simulink model "cyberAttack2"  (R2022b)
settings: Solver=VariableStepAuto  StartTime=0.0  StopTime=10  RelTol=1e-3
values from neighbouring files (symbols this model uses):
  attackTimeDelay = 0.1    [editor.m]
  attackTimeDelay1 = 0.1    [editor.m]
  CC_Kd = 0    [editor.m]
  CC_Ki = 150    [editor.m]
  CC_Kp = 0    [editor.m]
  enableObserver = 1    [editor.m]
  ICapacity_1 = 3    [editor.m]
  ICapacity_2 = 2    [editor.m]
  ILoadFinal = 2    [editor.m]
  ILoadInitial = 3    [editor.m]
  Kd = 4.6e-4    (= 0.00046)    [editor.m]
  Ki = 6.15    [editor.m]
  Kp = 0.1    [editor.m]
  N = 2.56e3    (= 2560)    [editor.m]
  Rij = 0.05    [editor.m]
  Rt = 0.2    [editor.m]
  timeOfAttack = 5    [editor.m]
  timeOfAttack1 = 5    [editor.m]
  tLoadChange = 6    [editor.m]
  Ts = 5e-5    (= 5e-05)    [editor.m]
  Vref = 40    [editor.m]
undefined symbols (not defined in the file or in its folder): Discrete, Time
libraries: fl_lib x54, nesl_utility_internal x30, slpidlib x8, simulink x4, ctrlSharedLib x4, ee_lib x4
(part 1 of 3)
settings Model: Creator=The MathWorks, Inc.  LastModifiedBy=bhuva

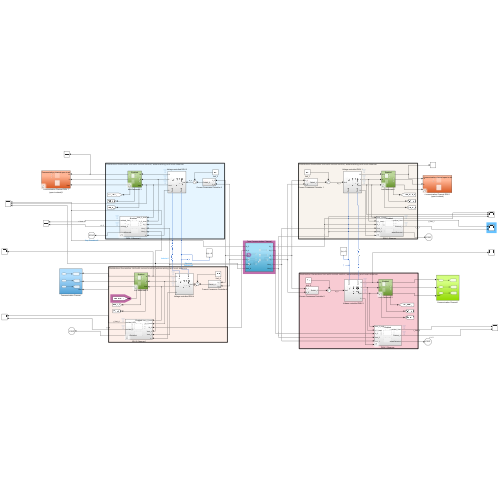
[thumbnail: Simulink's stored preview of the top-level diagram]
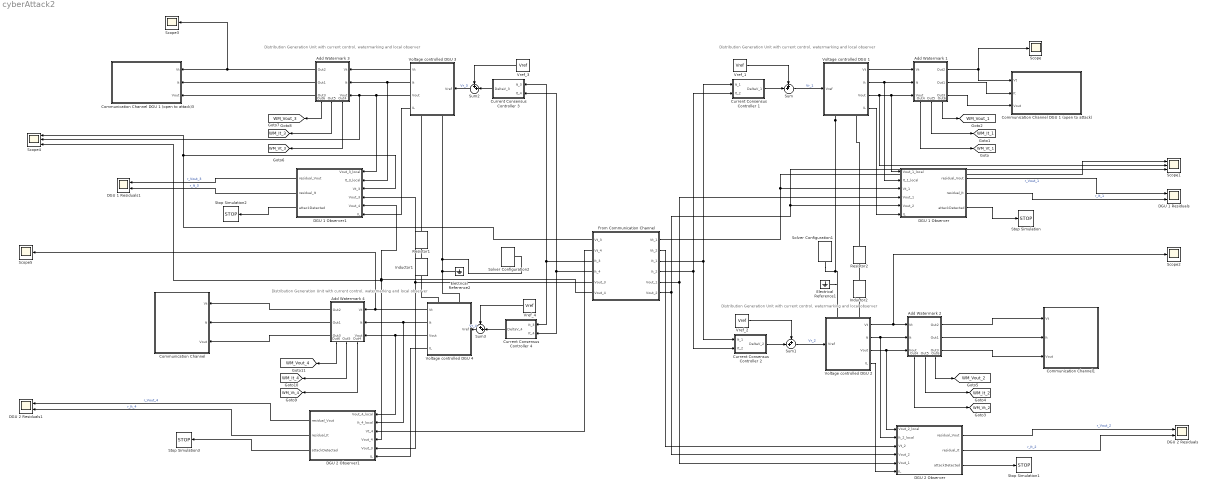
== system cyberAttack2 ==
  note: Distribution Generation Unit with current control, watermarking and local observer
  note: Distribution Generation Unit with current control, watermarking and local observer
  note: Distribution Generation Unit with current control, watermarking and local observer
  note: Distribution Generation Unit with current control, watermarking and local observer
  Add Watermark 1 : Subsystem  Variant=on  VariantControl=Choice
      settings: PortSchema="{\"entries\":[{\"content\":{\"sides\":[{\"content\":{\"connectorIds\":[\"In1\",\"In2\",\"In3\"]},\"type\":\"ConnectorPlacement.EquallySpacedRectSide\",\"uuid\":\"c94a7d77-0f2a-42c7-994c-f83d9f400b4a\"},{\"content\":{\"connectorIds\":[\"Out1\",\"Out2\",\"Out3\"],\"side\":\"RIGHT\"},\"type\":\"ConnectorPlacement.EquallySpacedRectSide\",\"uuid\":\"048bc904-366c-4deb-8d29-669922896a60\"},{\"content\":{\"connectorIds\":[],\"side\":\"TOP\"},\"type\":\"ConnectorPlacement.EquallySpacedRectSide\",\"uuid\":\"61856036-23df-49fc-9d48-72a95ac409b8\"},{\"content\":{\"connectorIds\":[\"Out4\",\"Out5\",\"Out6\"],\"side\":\"BOTTOM\"},\"type\":\"ConnectorPlacement.EquallySpacedRectSide\",\"uuid\":\"3c7882a6-545f-411e-a24e-2351be560f5c\"}]},\"type\":\"ConnectorPlacement.EquallySpacedConnector\",\"uuid\":\"82f313fb-6359-4167-9a1a-67611747de0f\"}],\"packageUris\":[\"http://schema.mathworks.com/mf0/Connector/R2020b\"],\"version\":\"1.0\"}"
  Add Watermark 2 : Subsystem  Variant=on  VariantControl=Choice
      settings: PortSchema="{\"entries\":[{\"content\":{\"sides\":[{\"content\":{\"connectorIds\":[\"In1\",\"In2\",\"In3\"]},\"type\":\"ConnectorPlacement.EquallySpacedRectSide\",\"uuid\":\"c94a7d77-0f2a-42c7-994c-f83d9f400b4a\"},{\"content\":{\"connectorIds\":[\"Out1\",\"Out2\",\"Out3\"],\"side\":\"RIGHT\"},\"type\":\"ConnectorPlacement.EquallySpacedRectSide\",\"uuid\":\"048bc904-366c-4deb-8d29-669922896a60\"},{\"content\":{\"connectorIds\":[],\"side\":\"TOP\"},\"type\":\"ConnectorPlacement.EquallySpacedRectSide\",\"uuid\":\"61856036-23df-49fc-9d48-72a95ac409b8\"},{\"content\":{\"connectorIds\":[\"Out4\",\"Out5\",\"Out6\"],\"side\":\"BOTTOM\"},\"type\":\"ConnectorPlacement.EquallySpacedRectSide\",\"uuid\":\"3c7882a6-545f-411e-a24e-2351be560f5c\"}]},\"type\":\"ConnectorPlacement.EquallySpacedConnector\",\"uuid\":\"82f313fb-6359-4167-9a1a-67611747de0f\"}],\"packageUris\":[\"http://schema.mathworks.com/mf0/Connector/R2020b\"],\"version\":\"1.0\"}"
  Add Watermark 3 : Subsystem  Variant=on  VariantControl=Choice
      settings: PortSchema="{\"entries\":[{\"content\":{\"sides\":[{\"content\":{\"connectorIds\":[\"In1\",\"In2\",\"In3\"]},\"type\":\"ConnectorPlacement.EquallySpacedRectSide\",\"uuid\":\"c94a7d77-0f2a-42c7-994c-f83d9f400b4a\"},{\"content\":{\"connectorIds\":[\"Out1\",\"Out2\",\"Out3\"],\"side\":\"RIGHT\"},\"type\":\"ConnectorPlacement.EquallySpacedRectSide\",\"uuid\":\"048bc904-366c-4deb-8d29-669922896a60\"},{\"content\":{\"connectorIds\":[],\"side\":\"TOP\"},\"type\":\"ConnectorPlacement.EquallySpacedRectSide\",\"uuid\":\"61856036-23df-49fc-9d48-72a95ac409b8\"},{\"content\":{\"connectorIds\":[\"Out4\",\"Out5\",\"Out6\"],\"side\":\"BOTTOM\"},\"type\":\"ConnectorPlacement.EquallySpacedRectSide\",\"uuid\":\"3c7882a6-545f-411e-a24e-2351be560f5c\"}]},\"type\":\"ConnectorPlacement.EquallySpacedConnector\",\"uuid\":\"82f313fb-6359-4167-9a1a-67611747de0f\"}],\"packageUris\":[\"http://schema.mathworks.com/mf0/Connector/R2020b\"],\"version\":\"1.0\"}"
  Add Watermark 4 : Subsystem  Variant=on  VariantControl=Choice
      settings: PortSchema="{\"entries\":[{\"content\":{\"sides\":[{\"content\":{\"connectorIds\":[\"In1\",\"In2\",\"In3\"]},\"type\":\"ConnectorPlacement.EquallySpacedRectSide\",\"uuid\":\"c94a7d77-0f2a-42c7-994c-f83d9f400b4a\"},{\"content\":{\"connectorIds\":[\"Out1\",\"Out2\",\"Out3\"],\"side\":\"RIGHT\"},\"type\":\"ConnectorPlacement.EquallySpacedRectSide\",\"uuid\":\"048bc904-366c-4deb-8d29-669922896a60\"},{\"content\":{\"connectorIds\":[],\"side\":\"TOP\"},\"type\":\"ConnectorPlacement.EquallySpacedRectSide\",\"uuid\":\"61856036-23df-49fc-9d48-72a95ac409b8\"},{\"content\":{\"connectorIds\":[\"Out4\",\"Out5\",\"Out6\"],\"side\":\"BOTTOM\"},\"type\":\"ConnectorPlacement.EquallySpacedRectSide\",\"uuid\":\"3c7882a6-545f-411e-a24e-2351be560f5c\"}]},\"type\":\"ConnectorPlacement.EquallySpacedConnector\",\"uuid\":\"82f313fb-6359-4167-9a1a-67611747de0f\"}],\"packageUris\":[\"http://schema.mathworks.com/mf0/Connector/R2020b\"],\"version\":\"1.0\"}"
  Communication Channel : Subsystem  VariantControl=enableAttack == 0
  Communication Channel DGU 1 (open to attack) : Subsystem  Variant=on  VariantControl=Choice
  Communication Channel DGU 1 (open to attack)3 : Subsystem  Variant=on  VariantControl=Choice
  Communication Channel1 : Subsystem  VariantControl=enableAttack1 == 0
  Current Consensus Controller 1 : Subsystem
  Current Consensus Controller 2 : Subsystem
  Current Consensus Controller 3 : Subsystem
  Current Consensus Controller 4 : Subsystem
  DGU 1 Observer : Subsystem  Variant=on  VariantControl=Choice
  DGU 1 Observer1 : Subsystem  Variant=on  VariantControl=Choice
  DGU 1 Residuals : Scope  NumInputPorts=2
  DGU 1 Residuals1 : Scope  NumInputPorts=2
  DGU 2 Observer : Subsystem  Variant=on  VariantControl=Choice
  DGU 2 Observer1 : Subsystem  Variant=on  VariantControl=Choice
  DGU 2 Residuals : Scope  NumInputPorts=2
  DGU 2 Residuals1 : Scope  NumInputPorts=2
  Electrical Reference1 : fl_lib/Electrical/Electrical Elements/Electrical Reference
  Electrical Reference2 : fl_lib/Electrical/Electrical Elements/Electrical Reference
  From Communication Channel : Subsystem
      settings: PortSchema="{\"entries\":[{\"content\":{\"sides\":[{\"content\":{\"connectorIds\":[\"Out7\",\"Out8\",\"Out9\",\"Out10\",\"Out11\",\"Out12\"]},\"type\":\"ConnectorPlacement.EquallySpacedRectSide\",\"uuid\":\"dab33db3-1f46-439d-aa3a-52ea6169c25e\"},{\"content\":{\"connectorIds\":[\"Out1\",\"Out2\",\"Out3\",\"Out4\",\"Out5\",\"Out6\"],\"side\":\"RIGHT\"},\"type\":\"ConnectorPlacement.EquallySpacedRectSide\",\"uuid\":\"8745bd78-99dc-4e19-8917-6cf580000ea6\"},{\"content\":{\"connectorIds\":[],\"side\":\"TOP\"},\"type\":\"ConnectorPlacement.EquallySpacedRectSide\",\"uuid\":\"a1611318-82ee-45f6-9432-dae462a0d549\"},{\"content\":{\"connectorIds\":[],\"side\":\"BOTTOM\"},\"type\":\"ConnectorPlacement.EquallySpacedRectSide\",\"uuid\":\"cb888c83-8f55-42f4-bbea-b76c8f1b8782\"}]},\"type\":\"ConnectorPlacement.EquallySpacedConnector\",\"uuid\":\"91a67cf2-7d11-4e60-8220-445a06462b3e\"}],\"packageUris\":[\"http://schema.mathworks.com/mf0/Connector/R2020b\"],\"version\":\"1.0\"}"
  Inductor1 : fl_lib/Electrical/Electrical Elements/Inductor  l=Lij H  r=0 Ohm  g=1e-9 1/Ohm  i_specify=off  i_priority=None  i=0 A  i_nominal_specify=off  i_nominal_unit=A  i_nominal_value=1  v_specify=off  v_priority=None  v=0 V  v_nominal_specify=off  v_nominal_unit=V  v_nominal_value=1  i_L_specify=off  i_L_priority=High  i_L=0 A  i_L_nominal_specify=off  i_L_nominal_unit=A  i_L_nominal_value=1
  Inductor2 : fl_lib/Electrical/Electrical Elements/Inductor  l=Lij H  r=0 Ohm  g=1e-9 1/Ohm  i_specify=off  i_priority=None  i=0 A  i_nominal_specify=off  i_nominal_unit=A  i_nominal_value=1  v_specify=off  v_priority=None  v=0 V  v_nominal_specify=off  v_nominal_unit=V  v_nominal_value=1  i_L_specify=off  i_L_priority=High  i_L=0 A  i_L_nominal_specify=off  i_L_nominal_unit=A  i_L_nominal_value=1
  Resistor1 : fl_lib/Electrical/Electrical Elements/Resistor  R=Rij Ohm  i_specify=off  i_priority=None  i=0 A  i_nominal_specify=off  i_nominal_unit=A  i_nominal_value=1  v_specify=off  v_priority=None  v=0 V  v_nominal_specify=off  v_nominal_unit=V  v_nominal_value=1
  Resistor2 : fl_lib/Electrical/Electrical Elements/Resistor  R=Rij Ohm  i_specify=off  i_priority=None  i=0 A  i_nominal_specify=off  i_nominal_unit=A  i_nominal_value=1  v_specify=off  v_priority=None  v=0 V  v_nominal_specify=off  v_nominal_unit=V  v_nominal_value=1
  Scope{,2..3,5} (4 alike) : Scope
  Scope1 : Scope  NumInputPorts=3
  Scope4 : Scope  NumInputPorts=3
  Solver Configuration1 : nesl_utility_internal/Solver Configuration  PhysicalDomain=network_engine_domain  SubClassName=solver  LeftPortType=input  RightPortType=generic  Tones=[]  Harmonics=[]  SimulateNoise=off  Profile=off  UseLocalSampling=off  EnableSwitchedLinearOptims=on  FrequencyDomain=off  UseCCode=off  RelTol=0.001  AbsTol=1e-06  MinStep=1e-09  ToWorkspace=off  RevertToSquareIcSolve=off  NumHomotopyIterations=100  PhasorMode=off  PhasorModeNumHarmonics=1  ConsistencySolver=NEWTON_FTOL  IndexReductionMethod=DerivativeReplacement  DoDC=off  ResidualTolerance=1e-9  ConsistencyTolSource=GLOBAL  ConsistencyAbsTol=0.001  ConsistencyRelTol=0.001  ConsistencyTolFactor=0.001  UseLocalSolver=on  LocalSolverChoice=NE_BACKWARD_EULER_ADVANCER  ResolveIndetEquations=on  FunctionEvalNumThread=1  LocalSolverSampleTime=Ts  DoFixedCost=on  MaxNonlinIter=3  MaxModeIter=2  ComputeImpulses=off  ImpulseIterations=2  LinearAlgebra=auto  LinearAlgebraNumThread=0  EquationFormulation=NE_TIME_EF  DelaysMemoryBudget=1024  AutomaticFiltering=on  FilteringTimeConstant=0.001  PartitionStorageMethod=AS_NEEDED  PartitionMemoryBudget=1024  PartitionMethod=FAST
  Solver Configuration2 : nesl_utility_internal/Solver Configuration  PhysicalDomain=network_engine_domain  SubClassName=solver  LeftPortType=input  RightPortType=generic  Tones=[]  Harmonics=[]  SimulateNoise=off  Profile=off  UseLocalSampling=off  EnableSwitchedLinearOptims=on  FrequencyDomain=off  UseCCode=off  RelTol=0.001  AbsTol=1e-06  MinStep=1e-09  ToWorkspace=off  RevertToSquareIcSolve=off  NumHomotopyIterations=100  PhasorMode=off  PhasorModeNumHarmonics=1  ConsistencySolver=NEWTON_FTOL  IndexReductionMethod=DerivativeReplacement  DoDC=off  ResidualTolerance=1e-9  ConsistencyTolSource=GLOBAL  ConsistencyAbsTol=0.001  ConsistencyRelTol=0.001  ConsistencyTolFactor=0.001  UseLocalSolver=on  LocalSolverChoice=NE_BACKWARD_EULER_ADVANCER  ResolveIndetEquations=on  FunctionEvalNumThread=1  LocalSolverSampleTime=Ts  DoFixedCost=on  MaxNonlinIter=3  MaxModeIter=2  ComputeImpulses=off  ImpulseIterations=2  LinearAlgebra=auto  LinearAlgebraNumThread=0  EquationFormulation=NE_TIME_EF  DelaysMemoryBudget=1024  AutomaticFiltering=on  FilteringTimeConstant=0.001  PartitionStorageMethod=AS_NEEDED  PartitionMemoryBudget=1024  PartitionMethod=FAST
  Stop Simulation{,1..3} (4 alike) : Stop
  Sum{,1..3} (4 alike) : Sum  Inputs=++|
  Voltage controlled DGU 1 : Subsystem
      settings: PortSchema="{\"entries\":[{\"content\":{\"sides\":[{\"content\":{\"connectorIds\":[]},\"type\":\"ConnectorPlacement.EquallySpacedRectSide\",\"uuid\":\"bd1f37b5-cace-475a-9319-df5dc175988c\"},{\"content\":{\"connectorIds\":[\"RConn1\",\"RConn2\"],\"side\":\"RIGHT\"},\"type\":\"ConnectorPlacement.EquallySpacedRectSide\",\"uuid\":\"6e9492d2-b492-4ddc-9bf9-c37fa50387fb\"},{\"content\":{\"connectorIds\":[\"Out1\",\"Out2\",\"Out3\",\"Out4\"],\"side\":\"TOP\"},\"type\":\"ConnectorPlacement.EquallySpacedRectSide\",\"uuid\":\"740d822e-a5fc-4d01-8f2e-7dd9c8c34700\"},{\"content\":{\"connectorIds\":[\"In1\"],\"side\":\"BOTTOM\"},\"type\":\"ConnectorPlacement.EquallySpacedRectSide\",\"uuid\":\"ce7350ec-18c7-472a-9669-30fb5abf65bf\"}]},\"type\":\"ConnectorPlacement.EquallySpacedConnector\",\"uuid\":\"15ef9329-fda5-41fa-bf9c-9b9fdaa2cf39\"}],\"packageUris\":[\"http://schema.mathworks.com/mf0/Connector/R2020b\"],\"version\":\"1.0\"}"
  Voltage controlled DGU 2 : Subsystem
      settings: PortSchema="{\"entries\":[{\"content\":{\"sides\":[{\"content\":{\"connectorIds\":[]},\"type\":\"ConnectorPlacement.EquallySpacedRectSide\",\"uuid\":\"bd1f37b5-cace-475a-9319-df5dc175988c\"},{\"content\":{\"connectorIds\":[\"RConn1\",\"RConn2\"],\"side\":\"RIGHT\"},\"type\":\"ConnectorPlacement.EquallySpacedRectSide\",\"uuid\":\"6e9492d2-b492-4ddc-9bf9-c37fa50387fb\"},{\"content\":{\"connectorIds\":[\"Out1\",\"Out2\",\"Out3\",\"Out4\"],\"side\":\"TOP\"},\"type\":\"ConnectorPlacement.EquallySpacedRectSide\",\"uuid\":\"740d822e-a5fc-4d01-8f2e-7dd9c8c34700\"},{\"content\":{\"connectorIds\":[\"In1\"],\"side\":\"BOTTOM\"},\"type\":\"ConnectorPlacement.EquallySpacedRectSide\",\"uuid\":\"ce7350ec-18c7-472a-9669-30fb5abf65bf\"}]},\"type\":\"ConnectorPlacement.EquallySpacedConnector\",\"uuid\":\"15ef9329-fda5-41fa-bf9c-9b9fdaa2cf39\"}],\"packageUris\":[\"http://schema.mathworks.com/mf0/Connector/R2020b\"],\"version\":\"1.0\"}"
  Voltage controlled DGU 3 : Subsystem
      settings: PortSchema="{\"entries\":[{\"content\":{\"sides\":[{\"content\":{\"connectorIds\":[]},\"type\":\"ConnectorPlacement.EquallySpacedRectSide\",\"uuid\":\"bd1f37b5-cace-475a-9319-df5dc175988c\"},{\"content\":{\"connectorIds\":[\"RConn1\",\"RConn2\"],\"side\":\"RIGHT\"},\"type\":\"ConnectorPlacement.EquallySpacedRectSide\",\"uuid\":\"6e9492d2-b492-4ddc-9bf9-c37fa50387fb\"},{\"content\":{\"connectorIds\":[\"Out1\",\"Out2\",\"Out3\",\"Out4\"],\"side\":\"TOP\"},\"type\":\"ConnectorPlacement.EquallySpacedRectSide\",\"uuid\":\"740d822e-a5fc-4d01-8f2e-7dd9c8c34700\"},{\"content\":{\"connectorIds\":[\"In1\"],\"side\":\"BOTTOM\"},\"type\":\"ConnectorPlacement.EquallySpacedRectSide\",\"uuid\":\"ce7350ec-18c7-472a-9669-30fb5abf65bf\"}]},\"type\":\"ConnectorPlacement.EquallySpacedConnector\",\"uuid\":\"15ef9329-fda5-41fa-bf9c-9b9fdaa2cf39\"}],\"packageUris\":[\"http://schema.mathworks.com/mf0/Connector/R2020b\"],\"version\":\"1.0\"}"
  Voltage controlled DGU 4 : Subsystem
      settings: PortSchema="{\"entries\":[{\"content\":{\"sides\":[{\"content\":{\"connectorIds\":[]},\"type\":\"ConnectorPlacement.EquallySpacedRectSide\",\"uuid\":\"bd1f37b5-cace-475a-9319-df5dc175988c\"},{\"content\":{\"connectorIds\":[\"RConn1\",\"RConn2\"],\"side\":\"RIGHT\"},\"type\":\"ConnectorPlacement.EquallySpacedRectSide\",\"uuid\":\"6e9492d2-b492-4ddc-9bf9-c37fa50387fb\"},{\"content\":{\"connectorIds\":[\"Out1\",\"Out2\",\"Out3\",\"Out4\"],\"side\":\"TOP\"},\"type\":\"ConnectorPlacement.EquallySpacedRectSide\",\"uuid\":\"740d822e-a5fc-4d01-8f2e-7dd9c8c34700\"},{\"content\":{\"connectorIds\":[\"In1\"],\"side\":\"BOTTOM\"},\"type\":\"ConnectorPlacement.EquallySpacedRectSide\",\"uuid\":\"ce7350ec-18c7-472a-9669-30fb5abf65bf\"}]},\"type\":\"ConnectorPlacement.EquallySpacedConnector\",\"uuid\":\"15ef9329-fda5-41fa-bf9c-9b9fdaa2cf39\"}],\"packageUris\":[\"http://schema.mathworks.com/mf0/Connector/R2020b\"],\"version\":\"1.0\"}"
  Vref_{1..4} (4 alike) : Constant  Value=Vref  SampleTime=Ts
  tag scope: WM_It_1=global, WM_It_2=global, WM_It_3=global, WM_It_4=global, WM_Vout_1=global, WM_Vout_2=global, WM_Vout_3=global, WM_Vout_4=global, WM_Vt_1=global, WM_Vt_2=global, WM_Vt_3=global, WM_Vt_4=global
  wires:
  Vref_1/1 -> Sum/1
  Sum/1 -> Voltage controlled DGU 1/1(Vref)  "Vr_1"
  Current Consensus Controller 1/1(DeltaV_1) -> Sum/2
  From Communication Channel/4(It_2) -> Current Consensus Controller 2/2(It_2), Current Consensus Controller 1/2(It_2)
  Voltage controlled DGU 1/3(Vout) -> Scope1/2, Add Watermark 1/3(Vout), DGU 1 Observer/1(Vout_1_local)
  Current Consensus Controller 2/1(DeltaV_2) -> Sum1/2
  Voltage controlled DGU 2/3(It) -> Add Watermark 2/2(It), DGU 2 Observer/2(It_2_local)
  Voltage controlled DGU 2/4(Vt) -> Scope2/1, Add Watermark 2/1(Vt)
  From Communication Channel/3(It_1) -> Current Consensus Controller 2/1(It_1), Current Consensus Controller 1/1(It_1)
  From Communication Channel/6(Vout_2) -> DGU 2 Observer/4(Vout_2), Scope1/3, DGU 1 Observer/5(Vout_2)
  Sum1/1 -> Voltage controlled DGU 2/1(Vref)  "Vr_2"
  From Communication Channel/5(Vout_1) -> DGU 2 Observer/5(Vout_1), DGU 1 Observer/4(Vout_1)
  Voltage controlled DGU 2/2(Vout) -> Add Watermark 2/3(Vout), DGU 2 Observer/1(Vout_2_local)
  Vref_2/1 -> Sum1/1
  Voltage controlled DGU 1/2(It) -> Add Watermark 1/2(It), DGU 1 Observer/2(It_1_local)
  DGU 2 Observer/3(attackDetected) -> Stop Simulation1/1
  From Communication Channel/1(Vt_1) -> Scope1/1, DGU 1 Observer/3(Vt_1)
  Voltage controlled DGU 1/4(IL) -> DGU 1 Observer/6(IL)
  From Communication Channel/2(Vt_2) -> DGU 2 Observer/3(Vt_2)
  Voltage controlled DGU 1/1(Vt) -> Add Watermark 1/1(Vt)
  Add Watermark 1/1(Out2) -> Communication Channel DGU 1 (open to attack)/1(Vt), Scope/1
  Add Watermark 1/2(Out1) -> Communication Channel DGU 1 (open to attack)/2(It)
  Add Watermark 1/3(Out3) -> Communication Channel DGU 1 (open to attack)/3(Vout)
  Add Watermark 1/4(Out4) -> [WM_Vt_1]
  Add Watermark 1/5(Out5) -> [WM_It_1]
  Add Watermark 1/6(Out6) -> [WM_Vout_1]
  DGU 1 Observer/1(residual_Vout) -> DGU 1 Residuals/1  "r_Vout_1"
  DGU 1 Observer/2(residual_It) -> DGU 1 Residuals/2  "r_It_1"
  DGU 1 Observer/3(attackDetected) -> Stop Simulation/1
  Voltage controlled DGU 2/1(IL) -> DGU 2 Observer/6(IL)
  DGU 2 Observer/1(residual_Vout) -> DGU 2 Residuals/1  "r_Vout_2"
  DGU 2 Observer/2(residual_It) -> DGU 2 Residuals/2  "r_It_2"
  Add Watermark 2/6(Out6) -> [WM_Vout_2]
  Add Watermark 2/5(Out5) -> [WM_It_2]
  Add Watermark 2/4(Out4) -> [WM_Vt_2]
  Add Watermark 2/1(Out2) -> Communication Channel1/1(Vt)
  Add Watermark 2/2(Out1) -> Communication Channel1/2(It)
  Add Watermark 2/3(Out3) -> Communication Channel1/3(Vout)
  From Communication Channel/11(Vout_3) -> DGU 2 Observer1/5(Vout_3), DGU 1 Observer1/4(Vout_3)
  DGU 1 Observer1/2(residual_It) -> DGU 1 Residuals1/2  "r_It_3"
  Voltage controlled DGU 4/1(IL) -> DGU 2 Observer1/6(IL)
  Add Watermark 3/4(Out4) -> [WM_Vt_3]
  Voltage controlled DGU 4/4(Vt) -> Scope5/1, Add Watermark 4/1(Vt)
  DGU 1 Observer1/3(attackDetected) -> Stop Simulation2/1
  From Communication Channel/9(It_3) -> Current Consensus Controller 3/1(It_3), Current Consensus Controller 4/1(It_3)
  Add Watermark 3/1(Out2) -> Scope3/1, Communication Channel DGU 1 (open to attack)3/1(Vt)
  DGU 2 Observer1/3(attackDetected) -> Stop Simulation3/1
  Sum3/1 -> Voltage controlled DGU 4/1(Vref)  "Vr_4"
  Vref_4/1 -> Sum3/1
  From Communication Channel/7(Vt_3) -> DGU 1 Observer1/3(Vt_3), Scope4/1
  Add Watermark 4/5(Out5) -> [WM_It_4]
  From Communication Channel/10(It_4) -> Current Consensus Controller 4/2(It_4), Current Consensus Controller 3/2(It_4)
  Voltage controlled DGU 4/2(Vout) -> Add Watermark 4/3(Vout), DGU 2 Observer1/1(Vout_4_local)
  Voltage controlled DGU 3/3(Vout) -> Add Watermark 3/3(Vout), Scope4/2, DGU 1 Observer1/1(Vout_3_local)
  From Communication Channel/8(Vt_4) -> DGU 2 Observer1/3(Vt_4)
  Voltage controlled DGU 3/4(IL) -> DGU 1 Observer1/6(IL)
  Current Consensus Controller 3/1(DeltaV_3) -> Sum2/2
  DGU 2 Observer1/2(residual_It) -> DGU 2 Residuals1/2  "r_It_4"
  Voltage controlled DGU 3/2(It) -> Add Watermark 3/2(It), DGU 1 Observer1/2(It_3_local)
  Vref_3/1 -> Sum2/1
  Add Watermark 4/4(Out4) -> [WM_Vt_4]
  Add Watermark 3/6(Out6) -> [WM_Vout_3]
  Voltage controlled DGU 4/3(It) -> Add Watermark 4/2(It), DGU 2 Observer1/2(It_4_local)
  DGU 2 Observer1/1(residual_Vout) -> DGU 2 Residuals1/1  "r_Vout_4"
  Current Consensus Controller 4/1(DeltaV_4) -> Sum3/2
  Voltage controlled DGU 3/1(Vt) -> Add Watermark 3/1(Vt)
  DGU 1 Observer1/1(residual_Vout) -> DGU 1 Residuals1/1  "r_Vout_3"
  From Communication Channel/12(Vout_4) -> DGU 1 Observer1/5(Vout_4), Scope4/3, DGU 2 Observer1/4(Vout_4)
  Add Watermark 4/6(Out6) -> [WM_Vout_4]
  Sum2/1 -> Voltage controlled DGU 3/1(Vref)  "Vr_3"
  Add Watermark 3/5(Out5) -> [WM_It_3]
  Add Watermark 4/1(Out2) -> Communication Channel/1(Vt)
  Add Watermark 4/2(Out1) -> Communication Channel/2(It)
  Add Watermark 4/3(Out3) -> Communication Channel/3(Vout)
  Add Watermark 3/2(Out1) -> Communication Channel DGU 1 (open to attack)3/2(It)
  Add Watermark 3/3(Out3) -> Communication Channel DGU 1 (open to attack)3/3(Vout)
  connections:
  Voltage controlled DGU 1/RConn2 -- Electrical Reference1/LConn1 -- Voltage controlled DGU 2/RConn2 -- Solver Configuration1/RConn1
  Inductor2/LConn1 -- Resistor2/RConn1
  Voltage controlled DGU 2/RConn1 -- Inductor2/RConn1
  Resistor2/LConn1 -- Voltage controlled DGU 1/RConn1
  Voltage controlled DGU 4/RConn2 -- Voltage controlled DGU 3/RConn2 -- Solver Configuration2/RConn1 -- Electrical Reference2/LConn1
  Inductor1/LConn1 -- Resistor1/RConn1
  Voltage controlled DGU 4/RConn1 -- Inductor1/RConn1
  Resistor1/LConn1 -- Voltage controlled DGU 3/RConn1

== system cyberAttack2/Add Watermark 1 ==
  Vt : Inport
  It : Inport  Port=2
  Vout : Inport  Port=3
  Disabled : Subsystem  VariantControl=enableWatermarking == 0
      settings: PortSchema="{\"entries\":[{\"content\":{\"sides\":[{\"content\":{\"connectorIds\":[\"In1\",\"In2\",\"In3\"]},\"type\":\"ConnectorPlacement.EquallySpacedRectSide\",\"uuid\":\"c94a7d77-0f2a-42c7-994c-f83d9f400b4a\"},{\"content\":{\"connectorIds\":[\"Out1\",\"Out2\",\"Out3\"],\"side\":\"RIGHT\"},\"type\":\"ConnectorPlacement.EquallySpacedRectSide\",\"uuid\":\"048bc904-366c-4deb-8d29-669922896a60\"},{\"content\":{\"connectorIds\":[],\"side\":\"TOP\"},\"type\":\"ConnectorPlacement.EquallySpacedRectSide\",\"uuid\":\"61856036-23df-49fc-9d48-72a95ac409b8\"},{\"content\":{\"connectorIds\":[\"Out4\",\"Out5\",\"Out6\"],\"side\":\"BOTTOM\"},\"type\":\"ConnectorPlacement.EquallySpacedRectSide\",\"uuid\":\"3c7882a6-545f-411e-a24e-2351be560f5c\"}]},\"type\":\"ConnectorPlacement.EquallySpacedConnector\",\"uuid\":\"82f313fb-6359-4167-9a1a-67611747de0f\"}],\"packageUris\":[\"http://schema.mathworks.com/mf0/Connector/R2020b\"],\"version\":\"1.0\"}"
  Enabled : Subsystem  VariantControl=enableWatermarking == 1
      settings: PortSchema="{\"entries\":[{\"content\":{\"sides\":[{\"content\":{\"connectorIds\":[\"In1\",\"In2\",\"In3\"]},\"type\":\"ConnectorPlacement.EquallySpacedRectSide\",\"uuid\":\"c94a7d77-0f2a-42c7-994c-f83d9f400b4a\"},{\"content\":{\"connectorIds\":[\"Out1\",\"Out2\",\"Out3\"],\"side\":\"RIGHT\"},\"type\":\"ConnectorPlacement.EquallySpacedRectSide\",\"uuid\":\"048bc904-366c-4deb-8d29-669922896a60\"},{\"content\":{\"connectorIds\":[],\"side\":\"TOP\"},\"type\":\"ConnectorPlacement.EquallySpacedRectSide\",\"uuid\":\"61856036-23df-49fc-9d48-72a95ac409b8\"},{\"content\":{\"connectorIds\":[\"Out4\",\"Out5\",\"Out6\"],\"side\":\"BOTTOM\"},\"type\":\"ConnectorPlacement.EquallySpacedRectSide\",\"uuid\":\"3c7882a6-545f-411e-a24e-2351be560f5c\"}]},\"type\":\"ConnectorPlacement.EquallySpacedConnector\",\"uuid\":\"82f313fb-6359-4167-9a1a-67611747de0f\"}],\"packageUris\":[\"http://schema.mathworks.com/mf0/Connector/R2020b\"],\"version\":\"1.0\"}"
  Out2 : Outport
  Out1 : Outport  Port=2
  Out3 : Outport  Port=3
  Out4 : Outport  Port=4
  Out5 : Outport  Port=5
  Out6 : Outport  Port=6

== system cyberAttack2/Add Watermark 2 ==
  Vt : Inport
  It : Inport  Port=2
  Vout : Inport  Port=3
  Disabled : Subsystem  VariantControl=enableWatermarking == 0
      settings: PortSchema="{\"entries\":[{\"content\":{\"sides\":[{\"content\":{\"connectorIds\":[\"In1\",\"In2\",\"In3\"]},\"type\":\"ConnectorPlacement.EquallySpacedRectSide\",\"uuid\":\"c94a7d77-0f2a-42c7-994c-f83d9f400b4a\"},{\"content\":{\"connectorIds\":[\"Out1\",\"Out2\",\"Out3\"],\"side\":\"RIGHT\"},\"type\":\"ConnectorPlacement.EquallySpacedRectSide\",\"uuid\":\"048bc904-366c-4deb-8d29-669922896a60\"},{\"content\":{\"connectorIds\":[],\"side\":\"TOP\"},\"type\":\"ConnectorPlacement.EquallySpacedRectSide\",\"uuid\":\"61856036-23df-49fc-9d48-72a95ac409b8\"},{\"content\":{\"connectorIds\":[\"Out4\",\"Out5\",\"Out6\"],\"side\":\"BOTTOM\"},\"type\":\"ConnectorPlacement.EquallySpacedRectSide\",\"uuid\":\"3c7882a6-545f-411e-a24e-2351be560f5c\"}]},\"type\":\"ConnectorPlacement.EquallySpacedConnector\",\"uuid\":\"82f313fb-6359-4167-9a1a-67611747de0f\"}],\"packageUris\":[\"http://schema.mathworks.com/mf0/Connector/R2020b\"],\"version\":\"1.0\"}"
  Enabled : Subsystem  VariantControl=enableWatermarking == 1
      settings: PortSchema="{\"entries\":[{\"content\":{\"sides\":[{\"content\":{\"connectorIds\":[\"In1\",\"In2\",\"In3\"]},\"type\":\"ConnectorPlacement.EquallySpacedRectSide\",\"uuid\":\"c94a7d77-0f2a-42c7-994c-f83d9f400b4a\"},{\"content\":{\"connectorIds\":[\"Out1\",\"Out2\",\"Out3\"],\"side\":\"RIGHT\"},\"type\":\"ConnectorPlacement.EquallySpacedRectSide\",\"uuid\":\"048bc904-366c-4deb-8d29-669922896a60\"},{\"content\":{\"connectorIds\":[],\"side\":\"TOP\"},\"type\":\"ConnectorPlacement.EquallySpacedRectSide\",\"uuid\":\"61856036-23df-49fc-9d48-72a95ac409b8\"},{\"content\":{\"connectorIds\":[\"Out4\",\"Out5\",\"Out6\"],\"side\":\"BOTTOM\"},\"type\":\"ConnectorPlacement.EquallySpacedRectSide\",\"uuid\":\"3c7882a6-545f-411e-a24e-2351be560f5c\"}]},\"type\":\"ConnectorPlacement.EquallySpacedConnector\",\"uuid\":\"82f313fb-6359-4167-9a1a-67611747de0f\"}],\"packageUris\":[\"http://schema.mathworks.com/mf0/Connector/R2020b\"],\"version\":\"1.0\"}"
  Out2 : Outport
  Out1 : Outport  Port=2
  Out3 : Outport  Port=3
  Out4 : Outport  Port=4
  Out5 : Outport  Port=5
  Out6 : Outport  Port=6

== system cyberAttack2/Add Watermark 3 ==
  Vt : Inport
  It : Inport  Port=2
  Vout : Inport  Port=3
  Disabled : Subsystem  VariantControl=enableWatermarking == 0
      settings: PortSchema="{\"entries\":[{\"content\":{\"sides\":[{\"content\":{\"connectorIds\":[\"In1\",\"In2\",\"In3\"]},\"type\":\"ConnectorPlacement.EquallySpacedRectSide\",\"uuid\":\"c94a7d77-0f2a-42c7-994c-f83d9f400b4a\"},{\"content\":{\"connectorIds\":[\"Out1\",\"Out2\",\"Out3\"],\"side\":\"RIGHT\"},\"type\":\"ConnectorPlacement.EquallySpacedRectSide\",\"uuid\":\"048bc904-366c-4deb-8d29-669922896a60\"},{\"content\":{\"connectorIds\":[],\"side\":\"TOP\"},\"type\":\"ConnectorPlacement.EquallySpacedRectSide\",\"uuid\":\"61856036-23df-49fc-9d48-72a95ac409b8\"},{\"content\":{\"connectorIds\":[\"Out4\",\"Out5\",\"Out6\"],\"side\":\"BOTTOM\"},\"type\":\"ConnectorPlacement.EquallySpacedRectSide\",\"uuid\":\"3c7882a6-545f-411e-a24e-2351be560f5c\"}]},\"type\":\"ConnectorPlacement.EquallySpacedConnector\",\"uuid\":\"82f313fb-6359-4167-9a1a-67611747de0f\"}],\"packageUris\":[\"http://schema.mathworks.com/mf0/Connector/R2020b\"],\"version\":\"1.0\"}"
  Enabled : Subsystem  VariantControl=enableWatermarking == 1
      settings: PortSchema="{\"entries\":[{\"content\":{\"sides\":[{\"content\":{\"connectorIds\":[\"In1\",\"In2\",\"In3\"]},\"type\":\"ConnectorPlacement.EquallySpacedRectSide\",\"uuid\":\"c94a7d77-0f2a-42c7-994c-f83d9f400b4a\"},{\"content\":{\"connectorIds\":[\"Out1\",\"Out2\",\"Out3\"],\"side\":\"RIGHT\"},\"type\":\"ConnectorPlacement.EquallySpacedRectSide\",\"uuid\":\"048bc904-366c-4deb-8d29-669922896a60\"},{\"content\":{\"connectorIds\":[],\"side\":\"TOP\"},\"type\":\"ConnectorPlacement.EquallySpacedRectSide\",\"uuid\":\"61856036-23df-49fc-9d48-72a95ac409b8\"},{\"content\":{\"connectorIds\":[\"Out4\",\"Out5\",\"Out6\"],\"side\":\"BOTTOM\"},\"type\":\"ConnectorPlacement.EquallySpacedRectSide\",\"uuid\":\"3c7882a6-545f-411e-a24e-2351be560f5c\"}]},\"type\":\"ConnectorPlacement.EquallySpacedConnector\",\"uuid\":\"82f313fb-6359-4167-9a1a-67611747de0f\"}],\"packageUris\":[\"http://schema.mathworks.com/mf0/Connector/R2020b\"],\"version\":\"1.0\"}"
  Out2 : Outport
  Out1 : Outport  Port=2
  Out3 : Outport  Port=3
  Out4 : Outport  Port=4
  Out5 : Outport  Port=5
  Out6 : Outport  Port=6

== system cyberAttack2/Add Watermark 4 ==
  Vt : Inport
  It : Inport  Port=2
  Vout : Inport  Port=3
  Disabled : Subsystem  VariantControl=enableWatermarking == 0
      settings: PortSchema="{\"entries\":[{\"content\":{\"sides\":[{\"content\":{\"connectorIds\":[\"In1\",\"In2\",\"In3\"]},\"type\":\"ConnectorPlacement.EquallySpacedRectSide\",\"uuid\":\"c94a7d77-0f2a-42c7-994c-f83d9f400b4a\"},{\"content\":{\"connectorIds\":[\"Out1\",\"Out2\",\"Out3\"],\"side\":\"RIGHT\"},\"type\":\"ConnectorPlacement.EquallySpacedRectSide\",\"uuid\":\"048bc904-366c-4deb-8d29-669922896a60\"},{\"content\":{\"connectorIds\":[],\"side\":\"TOP\"},\"type\":\"ConnectorPlacement.EquallySpacedRectSide\",\"uuid\":\"61856036-23df-49fc-9d48-72a95ac409b8\"},{\"content\":{\"connectorIds\":[\"Out4\",\"Out5\",\"Out6\"],\"side\":\"BOTTOM\"},\"type\":\"ConnectorPlacement.EquallySpacedRectSide\",\"uuid\":\"3c7882a6-545f-411e-a24e-2351be560f5c\"}]},\"type\":\"ConnectorPlacement.EquallySpacedConnector\",\"uuid\":\"82f313fb-6359-4167-9a1a-67611747de0f\"}],\"packageUris\":[\"http://schema.mathworks.com/mf0/Connector/R2020b\"],\"version\":\"1.0\"}"
  Enabled : Subsystem  VariantControl=enableWatermarking == 1
      settings: PortSchema="{\"entries\":[{\"content\":{\"sides\":[{\"content\":{\"connectorIds\":[\"In1\",\"In2\",\"In3\"]},\"type\":\"ConnectorPlacement.EquallySpacedRectSide\",\"uuid\":\"c94a7d77-0f2a-42c7-994c-f83d9f400b4a\"},{\"content\":{\"connectorIds\":[\"Out1\",\"Out2\",\"Out3\"],\"side\":\"RIGHT\"},\"type\":\"ConnectorPlacement.EquallySpacedRectSide\",\"uuid\":\"048bc904-366c-4deb-8d29-669922896a60\"},{\"content\":{\"connectorIds\":[],\"side\":\"TOP\"},\"type\":\"ConnectorPlacement.EquallySpacedRectSide\",\"uuid\":\"61856036-23df-49fc-9d48-72a95ac409b8\"},{\"content\":{\"connectorIds\":[\"Out4\",\"Out5\",\"Out6\"],\"side\":\"BOTTOM\"},\"type\":\"ConnectorPlacement.EquallySpacedRectSide\",\"uuid\":\"3c7882a6-545f-411e-a24e-2351be560f5c\"}]},\"type\":\"ConnectorPlacement.EquallySpacedConnector\",\"uuid\":\"82f313fb-6359-4167-9a1a-67611747de0f\"}],\"packageUris\":[\"http://schema.mathworks.com/mf0/Connector/R2020b\"],\"version\":\"1.0\"}"
  Out2 : Outport
  Out1 : Outport  Port=2
  Out3 : Outport  Port=3
  Out4 : Outport  Port=4
  Out5 : Outport  Port=5
  Out6 : Outport  Port=6

== system cyberAttack2/Communication Channel ==
  Vt : Inport
  It : Inport  Port=2
  Vout : Inport  Port=3
  tag scope: It_4=global, Vout_4=global, Vt_4=global
  wires:
  Vout/1 -> [Vout_4]
  It/1 -> [It_4]
  Vt/1 -> [Vt_4]

== system cyberAttack2/Communication Channel DGU 1 (open to attack) ==
  Vt : Inport
  It : Inport  Port=2
  Vout : Inport  Port=3
  Communication Channel : Subsystem  VariantControl=enableAttack == 0
  Communication channel open to attack : Subsystem  VariantControl=enableAttack == 1

== system cyberAttack2/Communication Channel DGU 1 (open to attack)3 ==
  Vt : Inport
  It : Inport  Port=2
  Vout : Inport  Port=3
  Communication Channel : Subsystem  VariantControl=enableAttack1 == 0
  Communication channel open to attack : Subsystem  VariantControl=enableAttack1 == 1

== system cyberAttack2/Communication Channel1 ==
  Vt : Inport
  It : Inport  Port=2
  Vout : Inport  Port=3
  tag scope: It_2=global, Vout_2=global, Vt_2=global
  wires:
  Vout/1 -> [Vout_2]
  It/1 -> [It_2]
  Vt/1 -> [Vt_2]

== system cyberAttack2/Current Consensus Controller 1 ==
  It_1 : Inport
  It_2 : Inport  Port=2
  Discrete PID Controller : slpidlib/PID Controller  Controller=PID  Form=Parallel  TimeDomain=Discrete-time  UseExternalTs=off  SampleTime=Ts  IntegratorMethod=Forward Euler  FilterMethod=Forward Euler  ControllerParametersSource=internal  P=CC_Kp  I=CC_Ki  UseKiTs=off  D=CC_Kd  N=1e4  UseFilter=on  TunerSelectOption=Transfer Function Based (PID Tuner App)  InitialConditionSource=internal  InitialConditionForIntegrator=0  InitialConditionForFilter=0  DifferentiatorICPrevScaledInput=0  ExternalReset=none  TrackingMode=off  Kt=1  LimitOutput=off  SatLimitsSource=internal  UpperSaturationLimit=inf  LowerSaturationLimit=-inf  LinearizeAsGain=off  AntiWindupMode=none  Kb=1  LimitIntegrator=off  UpperIntegratorSaturationLimit=inf  LowerIntegratorSaturationLimit=-inf  POutMin=[]  POutMax=[]  IOutMin=[]  IOutMax=[]  DOutMin=[]  DOutMax=[]  NOutMin=[]  NOutMax=[]  SumOutMin=[]  SumOutMax=[]  SaturationOutMin=[]  SaturationOutMax=[]  PParamMin=[]  PParamMax=[]  IParamMin=[]  IParamMax=[]  DParamMin=[]  DParamMax=[]  NParamMin=[]  NParamMax=[]  KbParamMin=[]  KbParamMax=[]  KtParamMin=[]  KtParamMax=[]  KbOutMin=[]  KbOutMax=[]  KtOutMin=[]  KtOutMax=[]  IntegratorOutMin=[]  IntegratorOutMax=[]  FilterOutMin=[]  FilterOutMax=[]  SumI1OutMin=[]  SumI1OutMax=[]  SumI2OutMin=[]  SumI2OutMax=[]  SumI3OutMin=[]  SumI3OutMax=[]  SumI4OutMin=[]  SumI4OutMax=[]  SumDOutMin=[]  SumDOutMax=[]  DifferentiatorOutMin=[]  DifferentiatorOutMax=[]  FilterDiffOutCoefMin=[]  FilterDiffOutCoefMax=[]  ReciprocalOutMin=[]  ReciprocalOutMax=[]  SumDenOutMin=[]  SumDenOutMax=[]  SumNumOutMin=[]  SumNumOutMax=[]  DivideOutMin=[]  DivideOutMax=[]  UdiffTsProdOutMin=[]  UdiffTsProdOutMax=[]  NTsProdOutMin=[]  NTsProdOutMax=[]  UintegralTsProdOutMin=[]  UintegralTsProdOutMax=[]  UngainTsProdOutMin=[]  UngainTsProdOutMax=[]  ClampingZeroOutDataTypeStr=Inherit: Inherit via back propagation  ClampingZeroOutMin=[]  ClampingZeroOutMax=[]  FilterDenConstantOutDataTypeStr=Inherit: Inherit via back propagation  FilterDenConstantOutMin=[]  FilterDenConstantOutMax=[]  PCopyOutDataTypeStr=Inherit: Inherit via back propagation  PCopyOutMin=[]  PCopyOutMax=[]  NCopyOutDataTypeStr=Inherit: Inherit via back propagation  NCopyOutMin=[]  NCopyOutMax=[]  IntegratorContinuousStateAttributes=''  IntegratorStateMustResolveToSignalObject=off  IntegratorRTWStateStorageClass=Auto  FilterContinuousStateAttributes=''  FilterStateMustResolveToSignalObject=off  FilterRTWStateStorageClass=Auto  ParallelPVariant=InternalParameters  IdealPVariant=Disabled  IVariant=InternalParameters  DVariant=InternalParameters  IntegratorVariant=Discrete  SatVariant=Disabled  AWVariant=Passthrough  PCopyVariant=Disabled  TRVariant=Disabled  FdbkBlocksVariant=Forward  IdealPFdbkVariant=Disabled  SatFdbkVariant=Disabled  DerivativeFilterVariant=ForwardEulerFilter  NVariant=InternalParameters  NCopyVariant=Disabled  FilterICVariant=InternalICsFilter  IntegratorICVariant=InternalICs  ExternalResetVariant=Disabled  TRSumVariant=Passthrough  SumFdbkVariant=Disabled  SumVariant=Sum_PID  TsampFilterVariant=InternalTs  TsampNgainVariant=Passthrough  TsampIntegralVariant=Passthrough  ExternalSaturationOutDataTypeStr=Inherit: Same as second input
      settings: LibrarySourceBlock=simulink/Discrete/Discrete PID Controller
  Gain7 : Gain  Gain=1/ICapacity_1
  Gain8 : Gain  Gain=1/ICapacity_2
  Sum : Sum  Inputs=-+|
  Sum1 : Sum  Inputs=-+|
  Sum4 : Sum  Inputs=|-+
  DeltaV_1 : Outport
  wires:
  Gain8/1 -> Sum4/2
  It_2/1 -> Sum1/2
  Gain7/1 -> Sum4/1
  Discrete PID Controller/1 -> DeltaV_1/1
  Sum/1 -> Gain7/1
  Sum1/1 -> Gain8/1
  It_1/1 -> Sum/2
  [WM_It_1] -> Sum/1
  [WM_It_2] -> Sum1/1
  Sum4/1 -> Discrete PID Controller/1

== system cyberAttack2/Current Consensus Controller 2 ==
  It_1 : Inport
  It_2 : Inport  Port=2
  Discrete PID Controller : slpidlib/PID Controller  Controller=PID  Form=Parallel  TimeDomain=Discrete-time  UseExternalTs=off  SampleTime=Ts  IntegratorMethod=Forward Euler  FilterMethod=Forward Euler  ControllerParametersSource=internal  P=CC_Kp  I=CC_Ki  UseKiTs=off  D=CC_Kd  N=1e4  UseFilter=on  TunerSelectOption=Transfer Function Based (PID Tuner App)  InitialConditionSource=internal  InitialConditionForIntegrator=0  InitialConditionForFilter=0  DifferentiatorICPrevScaledInput=0  ExternalReset=none  TrackingMode=off  Kt=1  LimitOutput=off  SatLimitsSource=internal  UpperSaturationLimit=inf  LowerSaturationLimit=-inf  LinearizeAsGain=off  AntiWindupMode=none  Kb=1  LimitIntegrator=off  UpperIntegratorSaturationLimit=inf  LowerIntegratorSaturationLimit=-inf  POutMin=[]  POutMax=[]  IOutMin=[]  IOutMax=[]  DOutMin=[]  DOutMax=[]  NOutMin=[]  NOutMax=[]  SumOutMin=[]  SumOutMax=[]  SaturationOutMin=[]  SaturationOutMax=[]  PParamMin=[]  PParamMax=[]  IParamMin=[]  IParamMax=[]  DParamMin=[]  DParamMax=[]  NParamMin=[]  NParamMax=[]  KbParamMin=[]  KbParamMax=[]  KtParamMin=[]  KtParamMax=[]  KbOutMin=[]  KbOutMax=[]  KtOutMin=[]  KtOutMax=[]  IntegratorOutMin=[]  IntegratorOutMax=[]  FilterOutMin=[]  FilterOutMax=[]  SumI1OutMin=[]  SumI1OutMax=[]  SumI2OutMin=[]  SumI2OutMax=[]  SumI3OutMin=[]  SumI3OutMax=[]  SumI4OutMin=[]  SumI4OutMax=[]  SumDOutMin=[]  SumDOutMax=[]  DifferentiatorOutMin=[]  DifferentiatorOutMax=[]  FilterDiffOutCoefMin=[]  FilterDiffOutCoefMax=[]  ReciprocalOutMin=[]  ReciprocalOutMax=[]  SumDenOutMin=[]  SumDenOutMax=[]  SumNumOutMin=[]  SumNumOutMax=[]  DivideOutMin=[]  DivideOutMax=[]  UdiffTsProdOutMin=[]  UdiffTsProdOutMax=[]  NTsProdOutMin=[]  NTsProdOutMax=[]  UintegralTsProdOutMin=[]  UintegralTsProdOutMax=[]  UngainTsProdOutMin=[]  UngainTsProdOutMax=[]  ClampingZeroOutDataTypeStr=Inherit: Inherit via back propagation  ClampingZeroOutMin=[]  ClampingZeroOutMax=[]  FilterDenConstantOutDataTypeStr=Inherit: Inherit via back propagation  FilterDenConstantOutMin=[]  FilterDenConstantOutMax=[]  PCopyOutDataTypeStr=Inherit: Inherit via back propagation  PCopyOutMin=[]  PCopyOutMax=[]  NCopyOutDataTypeStr=Inherit: Inherit via back propagation  NCopyOutMin=[]  NCopyOutMax=[]  IntegratorContinuousStateAttributes=''  IntegratorStateMustResolveToSignalObject=off  IntegratorRTWStateStorageClass=Auto  FilterContinuousStateAttributes=''  FilterStateMustResolveToSignalObject=off  FilterRTWStateStorageClass=Auto  ParallelPVariant=InternalParameters  IdealPVariant=Disabled  IVariant=InternalParameters  DVariant=InternalParameters  IntegratorVariant=Discrete  SatVariant=Disabled  AWVariant=Passthrough  PCopyVariant=Disabled  TRVariant=Disabled  FdbkBlocksVariant=Forward  IdealPFdbkVariant=Disabled  SatFdbkVariant=Disabled  DerivativeFilterVariant=ForwardEulerFilter  NVariant=InternalParameters  NCopyVariant=Disabled  FilterICVariant=InternalICsFilter  IntegratorICVariant=InternalICs  ExternalResetVariant=Disabled  TRSumVariant=Passthrough  SumFdbkVariant=Disabled  SumVariant=Sum_PID  TsampFilterVariant=InternalTs  TsampNgainVariant=Passthrough  TsampIntegralVariant=Passthrough  ExternalSaturationOutDataTypeStr=Inherit: Same as second input
      settings: LibrarySourceBlock=simulink/Discrete/Discrete PID Controller
  Gain7 : Gain  Gain=1/ICapacity_1
  Gain8 : Gain  Gain=1/ICapacity_2
  Sum : Sum  Inputs=-+|
  Sum1 : Sum  Inputs=-+|
  Sum4 : Sum  Inputs=|+-
  DeltaV_2 : Outport
  wires:
  Gain8/1 -> Sum4/2
  It_2/1 -> Sum1/2
  Sum4/1 -> Discrete PID Controller/1
  Gain7/1 -> Sum4/1
  Discrete PID Controller/1 -> DeltaV_2/1
  Sum/1 -> Gain7/1
  Sum1/1 -> Gain8/1
  It_1/1 -> Sum/2
  [WM_It_1] -> Sum/1
  [WM_It_2] -> Sum1/1

== system cyberAttack2/Current Consensus Controller 3 ==
  It_3 : Inport
  It_4 : Inport  Port=2
  Discrete PID Controller : slpidlib/PID Controller  Controller=PID  Form=Parallel  TimeDomain=Discrete-time  UseExternalTs=off  SampleTime=Ts  IntegratorMethod=Forward Euler  FilterMethod=Forward Euler  ControllerParametersSource=internal  P=CC_Kp  I=CC_Ki  UseKiTs=off  D=CC_Kd  N=1e4  UseFilter=on  TunerSelectOption=Transfer Function Based (PID Tuner App)  InitialConditionSource=internal  InitialConditionForIntegrator=0  InitialConditionForFilter=0  DifferentiatorICPrevScaledInput=0  ExternalReset=none  TrackingMode=off  Kt=1  LimitOutput=off  SatLimitsSource=internal  UpperSaturationLimit=inf  LowerSaturationLimit=-inf  LinearizeAsGain=off  AntiWindupMode=none  Kb=1  LimitIntegrator=off  UpperIntegratorSaturationLimit=inf  LowerIntegratorSaturationLimit=-inf  POutMin=[]  POutMax=[]  IOutMin=[]  IOutMax=[]  DOutMin=[]  DOutMax=[]  NOutMin=[]  NOutMax=[]  SumOutMin=[]  SumOutMax=[]  SaturationOutMin=[]  SaturationOutMax=[]  PParamMin=[]  PParamMax=[]  IParamMin=[]  IParamMax=[]  DParamMin=[]  DParamMax=[]  NParamMin=[]  NParamMax=[]  KbParamMin=[]  KbParamMax=[]  KtParamMin=[]  KtParamMax=[]  KbOutMin=[]  KbOutMax=[]  KtOutMin=[]  KtOutMax=[]  IntegratorOutMin=[]  IntegratorOutMax=[]  FilterOutMin=[]  FilterOutMax=[]  SumI1OutMin=[]  SumI1OutMax=[]  SumI2OutMin=[]  SumI2OutMax=[]  SumI3OutMin=[]  SumI3OutMax=[]  SumI4OutMin=[]  SumI4OutMax=[]  SumDOutMin=[]  SumDOutMax=[]  DifferentiatorOutMin=[]  DifferentiatorOutMax=[]  FilterDiffOutCoefMin=[]  FilterDiffOutCoefMax=[]  ReciprocalOutMin=[]  ReciprocalOutMax=[]  SumDenOutMin=[]  SumDenOutMax=[]  SumNumOutMin=[]  SumNumOutMax=[]  DivideOutMin=[]  DivideOutMax=[]  UdiffTsProdOutMin=[]  UdiffTsProdOutMax=[]  NTsProdOutMin=[]  NTsProdOutMax=[]  UintegralTsProdOutMin=[]  UintegralTsProdOutMax=[]  UngainTsProdOutMin=[]  UngainTsProdOutMax=[]  ClampingZeroOutDataTypeStr=Inherit: Inherit via back propagation  ClampingZeroOutMin=[]  ClampingZeroOutMax=[]  FilterDenConstantOutDataTypeStr=Inherit: Inherit via back propagation  FilterDenConstantOutMin=[]  FilterDenConstantOutMax=[]  PCopyOutDataTypeStr=Inherit: Inherit via back propagation  PCopyOutMin=[]  PCopyOutMax=[]  NCopyOutDataTypeStr=Inherit: Inherit via back propagation  NCopyOutMin=[]  NCopyOutMax=[]  IntegratorContinuousStateAttributes=''  IntegratorStateMustResolveToSignalObject=off  IntegratorRTWStateStorageClass=Auto  FilterContinuousStateAttributes=''  FilterStateMustResolveToSignalObject=off  FilterRTWStateStorageClass=Auto  ParallelPVariant=InternalParameters  IdealPVariant=Disabled  IVariant=InternalParameters  DVariant=InternalParameters  IntegratorVariant=Discrete  SatVariant=Disabled  AWVariant=Passthrough  PCopyVariant=Disabled  TRVariant=Disabled  FdbkBlocksVariant=Forward  IdealPFdbkVariant=Disabled  SatFdbkVariant=Disabled  DerivativeFilterVariant=ForwardEulerFilter  NVariant=InternalParameters  NCopyVariant=Disabled  FilterICVariant=InternalICsFilter  IntegratorICVariant=InternalICs  ExternalResetVariant=Disabled  TRSumVariant=Passthrough  SumFdbkVariant=Disabled  SumVariant=Sum_PID  TsampFilterVariant=InternalTs  TsampNgainVariant=Passthrough  TsampIntegralVariant=Passthrough  ExternalSaturationOutDataTypeStr=Inherit: Same as second input
      settings: LibrarySourceBlock=simulink/Discrete/Discrete PID Controller
  Gain7 : Gain  Gain=1/ICapacity_1
  Gain8 : Gain  Gain=1/ICapacity_2
  Sum : Sum  Inputs=-+|
  Sum1 : Sum  Inputs=-+|
  Sum4 : Sum  Inputs=|-+
  DeltaV_3 : Outport
  wires:
  Gain8/1 -> Sum4/2
  It_4/1 -> Sum1/2
  Gain7/1 -> Sum4/1
  Discrete PID Controller/1 -> DeltaV_3/1
  Sum/1 -> Gain7/1
  Sum1/1 -> Gain8/1
  It_3/1 -> Sum/2
  [WM_It_3] -> Sum/1
  [WM_It_4] -> Sum1/1
  Sum4/1 -> Discrete PID Controller/1

== system cyberAttack2/Current Consensus Controller 4 ==
  It_3 : Inport
  It_4 : Inport  Port=2
  Discrete PID Controller : slpidlib/PID Controller  Controller=PID  Form=Parallel  TimeDomain=Discrete-time  UseExternalTs=off  SampleTime=Ts  IntegratorMethod=Forward Euler  FilterMethod=Forward Euler  ControllerParametersSource=internal  P=CC_Kp  I=CC_Ki  UseKiTs=off  D=CC_Kd  N=1e4  UseFilter=on  TunerSelectOption=Transfer Function Based (PID Tuner App)  InitialConditionSource=internal  InitialConditionForIntegrator=0  InitialConditionForFilter=0  DifferentiatorICPrevScaledInput=0  ExternalReset=none  TrackingMode=off  Kt=1  LimitOutput=off  SatLimitsSource=internal  UpperSaturationLimit=inf  LowerSaturationLimit=-inf  LinearizeAsGain=off  AntiWindupMode=none  Kb=1  LimitIntegrator=off  UpperIntegratorSaturationLimit=inf  LowerIntegratorSaturationLimit=-inf  POutMin=[]  POutMax=[]  IOutMin=[]  IOutMax=[]  DOutMin=[]  DOutMax=[]  NOutMin=[]  NOutMax=[]  SumOutMin=[]  SumOutMax=[]  SaturationOutMin=[]  SaturationOutMax=[]  PParamMin=[]  PParamMax=[]  IParamMin=[]  IParamMax=[]  DParamMin=[]  DParamMax=[]  NParamMin=[]  NParamMax=[]  KbParamMin=[]  KbParamMax=[]  KtParamMin=[]  KtParamMax=[]  KbOutMin=[]  KbOutMax=[]  KtOutMin=[]  KtOutMax=[]  IntegratorOutMin=[]  IntegratorOutMax=[]  FilterOutMin=[]  FilterOutMax=[]  SumI1OutMin=[]  SumI1OutMax=[]  SumI2OutMin=[]  SumI2OutMax=[]  SumI3OutMin=[]  SumI3OutMax=[]  SumI4OutMin=[]  SumI4OutMax=[]  SumDOutMin=[]  SumDOutMax=[]  DifferentiatorOutMin=[]  DifferentiatorOutMax=[]  FilterDiffOutCoefMin=[]  FilterDiffOutCoefMax=[]  ReciprocalOutMin=[]  ReciprocalOutMax=[]  SumDenOutMin=[]  SumDenOutMax=[]  SumNumOutMin=[]  SumNumOutMax=[]  DivideOutMin=[]  DivideOutMax=[]  UdiffTsProdOutMin=[]  UdiffTsProdOutMax=[]  NTsProdOutMin=[]  NTsProdOutMax=[]  UintegralTsProdOutMin=[]  UintegralTsProdOutMax=[]  UngainTsProdOutMin=[]  UngainTsProdOutMax=[]  ClampingZeroOutDataTypeStr=Inherit: Inherit via back propagation  ClampingZeroOutMin=[]  ClampingZeroOutMax=[]  FilterDenConstantOutDataTypeStr=Inherit: Inherit via back propagation  FilterDenConstantOutMin=[]  FilterDenConstantOutMax=[]  PCopyOutDataTypeStr=Inherit: Inherit via back propagation  PCopyOutMin=[]  PCopyOutMax=[]  NCopyOutDataTypeStr=Inherit: Inherit via back propagation  NCopyOutMin=[]  NCopyOutMax=[]  IntegratorContinuousStateAttributes=''  IntegratorStateMustResolveToSignalObject=off  IntegratorRTWStateStorageClass=Auto  FilterContinuousStateAttributes=''  FilterStateMustResolveToSignalObject=off  FilterRTWStateStorageClass=Auto  ParallelPVariant=InternalParameters  IdealPVariant=Disabled  IVariant=InternalParameters  DVariant=InternalParameters  IntegratorVariant=Discrete  SatVariant=Disabled  AWVariant=Passthrough  PCopyVariant=Disabled  TRVariant=Disabled  FdbkBlocksVariant=Forward  IdealPFdbkVariant=Disabled  SatFdbkVariant=Disabled  DerivativeFilterVariant=ForwardEulerFilter  NVariant=InternalParameters  NCopyVariant=Disabled  FilterICVariant=InternalICsFilter  IntegratorICVariant=InternalICs  ExternalResetVariant=Disabled  TRSumVariant=Passthrough  SumFdbkVariant=Disabled  SumVariant=Sum_PID  TsampFilterVariant=InternalTs  TsampNgainVariant=Passthrough  TsampIntegralVariant=Passthrough  ExternalSaturationOutDataTypeStr=Inherit: Same as second input
      settings: LibrarySourceBlock=simulink/Discrete/Discrete PID Controller
  Gain7 : Gain  Gain=1/ICapacity_1
  Gain8 : Gain  Gain=1/ICapacity_2
  Sum : Sum  Inputs=-+|
  Sum1 : Sum  Inputs=-+|
  Sum4 : Sum  Inputs=|+-
  DeltaV_4 : Outport
  wires:
  Gain8/1 -> Sum4/2
  It_4/1 -> Sum1/2
  Sum4/1 -> Discrete PID Controller/1
  Gain7/1 -> Sum4/1
  Discrete PID Controller/1 -> DeltaV_4/1
  Sum/1 -> Gain7/1
  Sum1/1 -> Gain8/1
  It_3/1 -> Sum/2
  [WM_It_3] -> Sum/1
  [WM_It_4] -> Sum1/1

== system cyberAttack2/DGU 1 Observer ==
  Vout_1_local : Inport
  It_1_local : Inport  Port=2
  Vt_1 : Inport  Port=3
  Vout_1 : Inport  Port=4
  Vout_2 : Inport  Port=5
  IL : Inport  Port=6
  Disabled : Subsystem  VariantControl=enableObserver == 0
      settings: PortSchema="{\"entries\":[{\"content\":{\"sides\":[{\"content\":{\"connectorIds\":[\"In1\",\"In2\",\"In3\",\"In4\"]},\"type\":\"ConnectorPlacement.EquallySpacedRectSide\",\"uuid\":\"1fcbc3c4-c380-448d-a7a8-357aa057b5ad\"},{\"content\":{\"connectorIds\":[\"Out1\",\"Out2\",\"Out3\"],\"side\":\"RIGHT\"},\"type\":\"ConnectorPlacement.EquallySpacedRectSide\",\"uuid\":\"7cbaad62-7890-4094-8ace-3159eca04825\"},{\"content\":{\"connectorIds\":[\"In5\",\"In6\"],\"side\":\"TOP\"},\"type\":\"ConnectorPlacement.EquallySpacedRectSide\",\"uuid\":\"f6c34017-9df2-4479-96e0-d67eb53c1d2d\"}]},\"type\":\"ConnectorPlacement.EquallySpacedConnector\",\"uuid\":\"f0a4a9b8-ed06-4c65-915f-6b202d377626\"}],\"packageUris\":[\"http://schema.mathworks.com/mf0/Connector/R2020b\"],\"version\":\"1.0\"}"
  Enabled : Subsystem  VariantControl=enableObserver == 1
      settings: PortSchema="{\"entries\":[{\"content\":{\"sides\":[{\"content\":{\"connectorIds\":[\"In1\",\"In2\",\"In3\",\"In4\"]},\"type\":\"ConnectorPlacement.EquallySpacedRectSide\",\"uuid\":\"1fcbc3c4-c380-448d-a7a8-357aa057b5ad\"},{\"content\":{\"connectorIds\":[\"Out1\",\"Out2\",\"Out3\"],\"side\":\"RIGHT\"},\"type\":\"ConnectorPlacement.EquallySpacedRectSide\",\"uuid\":\"7cbaad62-7890-4094-8ace-3159eca04825\"},{\"content\":{\"connectorIds\":[\"In5\",\"In6\"],\"side\":\"TOP\"},\"type\":\"ConnectorPlacement.EquallySpacedRectSide\",\"uuid\":\"f6c34017-9df2-4479-96e0-d67eb53c1d2d\"}]},\"type\":\"ConnectorPlacement.EquallySpacedConnector\",\"uuid\":\"f0a4a9b8-ed06-4c65-915f-6b202d377626\"}],\"packageUris\":[\"http://schema.mathworks.com/mf0/Connector/R2020b\"],\"version\":\"1.0\"}"
  residual_Vout : Outport
  residual_It : Outport  Port=2
  attackDetected : Outport  Port=3
